simulink model "final_control_model08t02_02"  (R2014b)
settings: Solver=ode3  StartTime=0.0  StopTime=1200  FixedStep=0.1  RelTol=1e-3
libraries: simulink x2
settings Model: PauseTimes=0  SnapshotBufferSize=100  Creator=Administrator  LastModifiedBy=Administrator

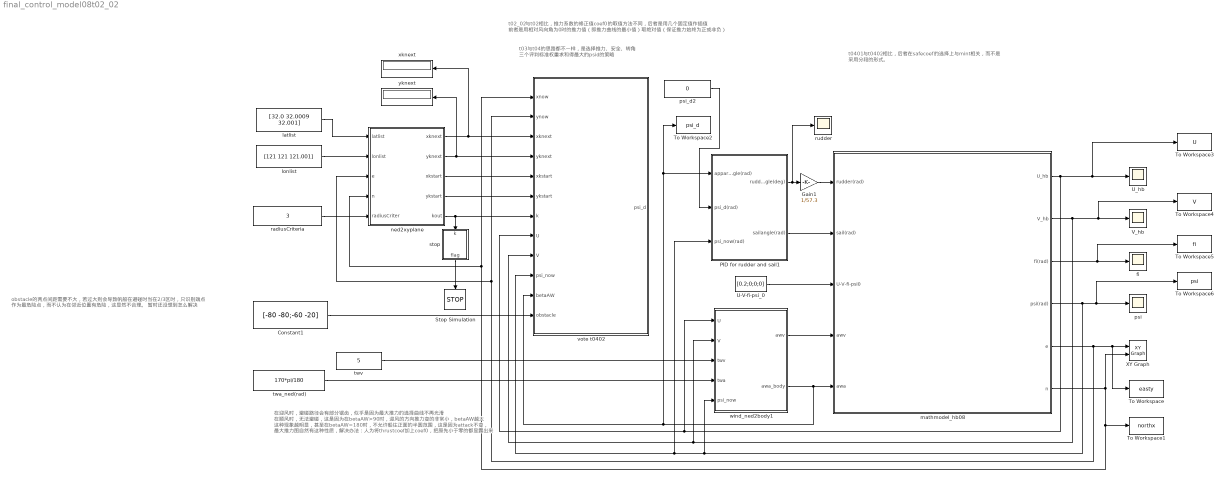
== system final_control_model08t02_02 ==
  note: obstacle的两点间距需要不大，若过大则会导致帆船在避碰时当在2/3区时，只识别端点
      | 作为最危险点，而不认为在邻近位置有危险，这显然不合理。
      | 暂时还没想到怎么解决
  note: t02_02与t02相比，推力系数的修正值coef0的取值方法不同，后者是用几个固定值作插值
      | 前者是用相对风向角为0时的推力值（即推力曲线的最小值）取绝对值（保证推力始终为正或非负）
  note: t0401与t0402相比，后者在safecoef的选择上与mint相关，而不是
      | 采用分段的形式。
  note: 在迎风时，避碰路径会有部分锯齿，似乎是因为最大推力的选择曲线不再光滑
      | 在顺风时，无法避碰，这是因为在betaAW>90时，迎风的方向推力变的非常小，betaAW越大
      | 这种现象越明显，甚至在betaAW=180时，不允许船往正面的半圆范围，这是因为attack不变，
      | 最大推力图自然有这种性质，解决办法：人为将thrustcoef加上coef0，把原先小于零的都显露出来
  note: t03与t04的思路都不一样，是选择推力、安全、转角
      | 三个评判标准权重求和得最大的psid的策略
  Constant1 : Constant  Value=[-80 -80;-60 -20]
  Gain1 : Gain  Gain=1/57.3
  PID for rudder and sail1 : Subsystem
  Stop Simulation : Stop
  To Workspace : ToWorkspace  VariableName=easty  SaveFormat=Timeseries  SampleTime=-1
  To Workspace1 : ToWorkspace  VariableName=northx  SaveFormat=Timeseries  SampleTime=-1
  To Workspace2 : ToWorkspace  VariableName=psi_d  SaveFormat=Timeseries  SampleTime=-1
  To Workspace3 : ToWorkspace  VariableName=U  SaveFormat=Timeseries  SampleTime=-1
  To Workspace4 : ToWorkspace  VariableName=V  SaveFormat=Timeseries  SampleTime=-1
  To Workspace5 : ToWorkspace  VariableName=fi  SaveFormat=Timeseries  SampleTime=-1
  To Workspace6 : ToWorkspace  VariableName=psi  SaveFormat=Timeseries  SampleTime=-1
  U-V-fi-psi_0 : Constant  Value=[0.2;0;0;0]
  U_hb : Scope
      settings: YMin=-0.045  YMax=0  SaveName=ScopeData2
  V_hb : Scope
      settings: YMin=-0.1  YMax=0.1
  XY Graph : simulink/Sinks/XY Graph  xmin=-050  xmax=150  ymin=-50  ymax=150  st=-1
  fi : Scope
      settings: YMin=-0.2  YMax=0.25
  "latlist " : Constant  Value=[32.0 32.0009 32.001]
  lonlist : Constant  Value=[121 121 121.001]
  "mathmodel_hb08 " : Subsystem
  ned2xyplane : Subsystem
  "psi " : Scope
      settings: YMin=-4  YMax=4  SaveName=ScopeData3
  psi_d2 : Constant  Value=0
  radiusCriteria : Constant  Value=3
  rudder : Scope
      settings: YMin=-40  YMax=40  SaveName=ScopeData4
  stop : MATLAB Function  TreatAsAtomicUnit=on
  twa_ned(rad) : Constant  Value=170*pi/180
  twv : Constant  Value=5
  vote t0402 : MATLAB Function  TreatAsAtomicUnit=on
  wind_ned2body1 : Subsystem
  xknext : Display
  yknext : Display
  wires:
  U-V-fi-psi_0/1 -> "mathmodel_hb08 "/3(U-V-fi-psi0)
  "mathmodel_hb08 "/1(U_hb) -> To Workspace3/1, U_hb/1, vote t0402/8(U), wind_ned2body1/1(U)
  "mathmodel_hb08 "/2(V_hb) -> vote t0402/9(V), wind_ned2body1/2(V), To Workspace4/1, V_hb/1
  "mathmodel_hb08 "/3(fi(rad)) -> To Workspace5/1, fi/1
  "mathmodel_hb08 "/4(psi(rad)) -> To Workspace6/1, "psi "/1, PID for rudder and sail1/3(psi_now(rad)), vote t0402/10(psi_now), wind_ned2body1/5(psi_now)
  PID for rudder and sail1/1(rudderangle(deg)) -> rudder/1, Gain1/1
  PID for rudder and sail1/2(sailangle(rad)) -> "mathmodel_hb08 "/2(sail(rad))
  Gain1/1 -> "mathmodel_hb08 "/1(rudder(rad))
  "mathmodel_hb08 "/5(e) -> To Workspace/1, XY Graph/1, vote t0402/2(ynow), ned2xyplane/3(e)
  "mathmodel_hb08 "/6(n) -> To Workspace1/1, ned2xyplane/4(n), vote t0402/1(xnow), XY Graph/2
  wind_ned2body1/2(awa_body) -> "mathmodel_hb08 "/5(awa), To Workspace2/1, PID for rudder and sail1/1(apparent wind angle(rad)), vote t0402/11(betaAW)
  wind_ned2body1/1(awv) -> "mathmodel_hb08 "/4(awv)
  twv/1 -> wind_ned2body1/3(twv)
  twa_ned(rad)/1 -> wind_ned2body1/4(twa)
  Constant1/1 -> vote t0402/12(obstacle)
  ned2xyplane/2(yknext) -> yknext/1, vote t0402/4(yknext)
  ned2xyplane/1(xknext) -> xknext/1, vote t0402/3(xknext)
  "latlist "/1 -> ned2xyplane/1(latlist)
  lonlist/1 -> ned2xyplane/2(lonlist)
  radiusCriteria/1 -> ned2xyplane/5(radiusCriter)
  ned2xyplane/3(xkstart) -> vote t0402/5(xkstart)
  ned2xyplane/4(ykstart) -> vote t0402/6(ykstart)
  ned2xyplane/5(kout) -> stop/1(k), vote t0402/7(k)
  stop/1(flag) -> Stop Simulation/1
  psi_d2/1 -> PID for rudder and sail1/2(psi_d(rad))

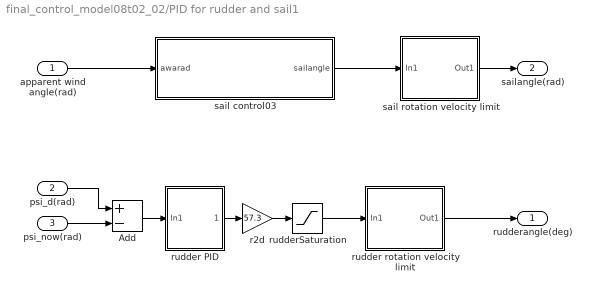
== system final_control_model08t02_02/PID for rudder and sail1 ==
  apparent wind angle(rad) : Inport
  psi_d(rad) : Inport  Port=2
  psi_now(rad) : Inport  Port=3
  Add : Sum  Inputs=+-
  r2d : Gain  Gain=57.3
  rudder PID : Subsystem
  rudder rotation velocity limit : Subsystem
  rudderSaturation : Saturate  UpperLimit=35  LowerLimit=-35
  sail control03 : MATLAB Function  TreatAsAtomicUnit=on
  sail rotation velocity limit : Subsystem
  rudderangle(deg) : Outport
  sailangle(rad) : Outport  Port=2
  wires:
  apparent wind angle(rad)/1 -> sail control03/1(awarad)
  psi_now(rad)/1 -> Add/2
  psi_d(rad)/1 -> Add/1
  Add/1 -> rudder PID/1(In1)
  rudder PID/1(rudder) -> r2d/1
  r2d/1 -> rudderSaturation/1
  rudderSaturation/1 -> rudder rotation velocity limit/1(In1)
  rudder rotation velocity limit/1(Out1) -> rudderangle(deg)/1
  sail control03/1(sailangle) -> sail rotation velocity limit/1(In1)
  sail rotation velocity limit/1(Out1) -> sailangle(rad)/1

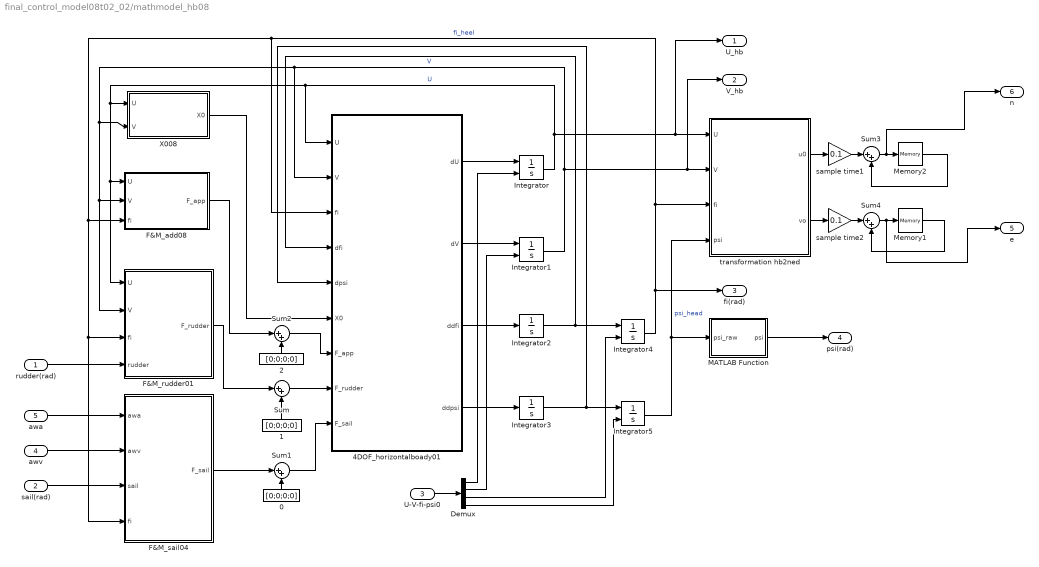
== system final_control_model08t02_02/mathmodel_hb08  ==
  rudder(rad) : Inport
  sail(rad) : Inport  Port=2
  U-V-fi-psi0 : Inport  Port=3
  awv : Inport  Port=4
  awa : Inport  Port=5
  0 : Constant  Value=[0;0;0;0]
  1 : Constant  Value=[0;0;0;0]
  2 : Constant  Value=[0;0;0;0]
  4DOF_horizontalboady01 : MATLAB Function  TreatAsAtomicUnit=on
  Demux : Demux
  F&M_add08 : MATLAB Function  TreatAsAtomicUnit=on
  F&M_rudder01 : MATLAB Function  TreatAsAtomicUnit=on
  F&M_sail04 : MATLAB Function  TreatAsAtomicUnit=on
  Integrator{,1,4..5} (4 alike) : Integrator  InitialConditionSource=external
  Integrator2 : Integrator
  Integrator3 : Integrator
  MATLAB Function : MATLAB Function  TreatAsAtomicUnit=on
  Memory1 : Memory  InheritSampleTime=on
  Memory2 : Memory  InheritSampleTime=on
  Sum{,1..4} (5 alike) : Sum  Inputs=|++
  X008 : MATLAB Function  TreatAsAtomicUnit=on
  sample time1 : Gain  Gain=0.1
  sample time2 : Gain  Gain=0.1
  transformation hb2ned : MATLAB Function  TreatAsAtomicUnit=on
  U_hb : Outport
  V_hb : Outport  Port=2
  fi(rad) : Outport  Port=3
  psi(rad) : Outport  Port=4
  e : Outport  Port=5
  n : Outport  Port=6
  wires:
  Integrator2/1 -> Integrator4/1, 4DOF_horizontalboady01/4(dfi)
  Integrator4/1 -> fi(rad)/1, transformation hb2ned/3(fi), 4DOF_horizontalboady01/3(fi), F&M_add08/3(fi), F&M_rudder01/3(fi), F&M_sail04/4(fi)  "fi_heel"
  4DOF_horizontalboady01/2(dV) -> Integrator1/1
  Integrator3/1 -> Integrator5/1, 4DOF_horizontalboady01/5(dpsi)
  4DOF_horizontalboady01/3(ddfi) -> Integrator2/1
  Integrator5/1 -> transformation hb2ned/4(psi), MATLAB Function/1(psi_raw)  "psi_head"
  X008/1(X0) -> 4DOF_horizontalboady01/6(X0)
  4DOF_horizontalboady01/1(dU) -> Integrator/1
  4DOF_horizontalboady01/4(ddpsi) -> Integrator3/1
  Integrator/1 -> 4DOF_horizontalboady01/1(U), F&M_add08/1(U), F&M_rudder01/1(U), X008/1(U), U_hb/1, transformation hb2ned/1(U)  "U"
  Integrator1/1 -> F&M_add08/2(V), F&M_rudder01/2(V), X008/2(V), 4DOF_horizontalboady01/2(V), V_hb/1, transformation hb2ned/2(V)  "V"
  Demux/3 -> Integrator4/2
  awa/1 -> F&M_sail04/1(awa)
  Demux/1 -> Integrator/2
  sail(rad)/1 -> F&M_sail04/3(sail)
  awv/1 -> F&M_sail04/2(awv)
  rudder(rad)/1 -> F&M_rudder01/4(rudder)
  Demux/4 -> Integrator5/2
  Demux/2 -> Integrator1/2
  F&M_rudder01/1(F_rudder) -> Sum/1
  F&M_add08/1(F_app) -> Sum2/1
  sample time2/1 -> Sum4/1
  Sum3/1 -> Memory2/1, n/1
  Memory2/1 -> Sum3/2
  F&M_sail04/1(F_sail) -> Sum1/1
  Sum2/1 -> 4DOF_horizontalboady01/7(F_app)
  transformation hb2ned/2(vo) -> sample time2/1
  Memory1/1 -> Sum4/2
  Sum4/1 -> e/1, Memory1/1
  U-V-fi-psi0/1 -> Demux/1
  2/1 -> Sum2/2
  Sum/1 -> 4DOF_horizontalboady01/8(F_rudder)
  sample time1/1 -> Sum3/1
  1/1 -> Sum/2
  0/1 -> Sum1/2
  transformation hb2ned/1(u0) -> sample time1/1
  Sum1/1 -> 4DOF_horizontalboady01/9(F_sail)
  MATLAB Function/1(psi) -> psi(rad)/1

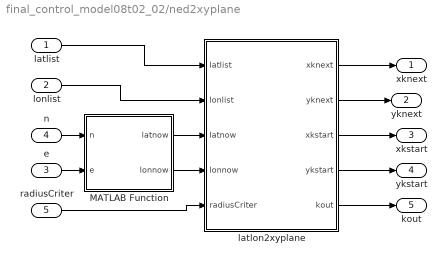
== system final_control_model08t02_02/ned2xyplane ==
  latlist : Inport
  lonlist : Inport  Port=2
  e : Inport  Port=3
  n : Inport  Port=4
  radiusCriter : Inport  Port=5
  MATLAB Function : MATLAB Function  TreatAsAtomicUnit=on
  latlon2xyplane : MATLAB Function  TreatAsAtomicUnit=on
  xknext : Outport
  yknext : Outport  Port=2
  xkstart : Outport  Port=3
  ykstart : Outport  Port=4
  kout : Outport  Port=5
  wires:
  latlon2xyplane/2(yknext) -> yknext/1
  latlist/1 -> latlon2xyplane/1(latlist)
  lonlist/1 -> latlon2xyplane/2(lonlist)
  MATLAB Function/1(latnow) -> latlon2xyplane/3(latnow)
  latlon2xyplane/1(xknext) -> xknext/1
  radiusCriter/1 -> latlon2xyplane/5(radiusCriter)
  latlon2xyplane/3(xkstart) -> xkstart/1
  latlon2xyplane/4(ykstart) -> ykstart/1
  latlon2xyplane/5(kout) -> kout/1
  MATLAB Function/2(lonnow) -> latlon2xyplane/4(lonnow)
  e/1 -> MATLAB Function/2(e)
  n/1 -> MATLAB Function/1(n)

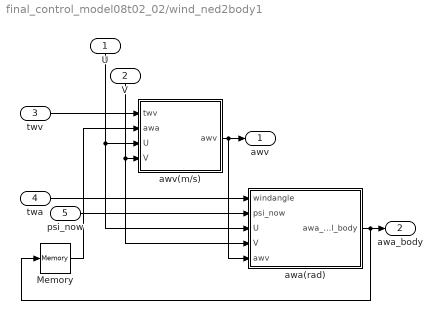
== system final_control_model08t02_02/wind_ned2body1 ==
  U : Inport
  V : Inport  Port=2
  twv : Inport  Port=3
  twa : Inport  Port=4
  psi_now : Inport  Port=5
  Memory : Memory
  awa(rad) : MATLAB Function  TreatAsAtomicUnit=on
  awv(m/s) : MATLAB Function  TreatAsAtomicUnit=on
  awv : Outport
  awa_body : Outport  Port=2
  wires:
  twa/1 -> awa(rad)/1(windangle)
  Memory/1 -> awv(m/s)/2(awa)
  twv/1 -> awv(m/s)/1(twv)
  V/1 -> awa(rad)/4(V), awv(m/s)/4(V)
  awv(m/s)/1(awv) -> awa(rad)/5(awv), awv/1
  psi_now/1 -> awa(rad)/2(psi_now)
  U/1 -> awa(rad)/3(U), awv(m/s)/3(U)
  awa(rad)/1(awa_cal_body) -> Memory/1, awa_body/1

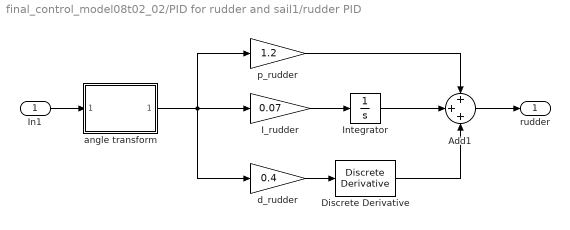
== system final_control_model08t02_02/PID for rudder and sail1/rudder PID ==
  In1 : Inport
  Add1 : Sum  Inputs=+++
  Discrete Derivative : simulink/Discrete/Discrete Derivative  gainval=1.0  ICPrevScaledInput=0.0  InputProcessing=Inherited  OutMin=[]  OutMax=[]  OutDataType=fixdt(1, 16)  OutScaling=2^-10  DoSatur=off
  I_rudder : Gain  Gain=0.07
  Integrator : Integrator
  angle transform : MATLAB Function  TreatAsAtomicUnit=on
  d_rudder : Gain  Gain=0.4
  p_rudder : Gain  Gain=1.2
  rudder : Outport
  wires:
  Integrator/1 -> Add1/2
  Discrete Derivative/1 -> Add1/3
  p_rudder/1 -> Add1/1
  d_rudder/1 -> Discrete Derivative/1
  angle transform/1(delta_pid) -> p_rudder/1, d_rudder/1, I_rudder/1
  In1/1 -> angle transform/1(delta_psi)
  I_rudder/1 -> Integrator/1
  Add1/1 -> rudder/1

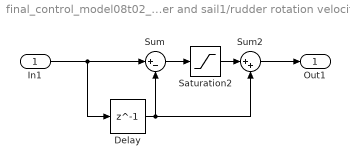
== system final_control_model08t02_02/PID for rudder and sail1/rudder rotation velocity limit ==
  In1 : Inport
  Delay : Delay  DelayLength=1  InitialCondition=0
  Saturation2 : Saturate  UpperLimit=4  LowerLimit=-4
  Sum : Sum  Inputs=|+-
  Sum2 : Sum  Inputs=|++
  Out1 : Outport
  wires:
  In1/1 -> Delay/1, Sum/1
  Sum2/1 -> Out1/1
  Saturation2/1 -> Sum2/1
  Sum/1 -> Saturation2/1
  Delay/1 -> Sum/2, Sum2/2

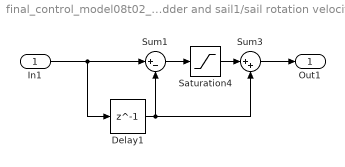
== system final_control_model08t02_02/PID for rudder and sail1/sail rotation velocity limit ==
  In1 : Inport
  Delay1 : Delay  DelayLength=1  InitialCondition=0
  Saturation4 : Saturate  UpperLimit=4  LowerLimit=-4
  Sum1 : Sum  Inputs=|+-
  Sum3 : Sum  Inputs=|++
  Out1 : Outport
  wires:
  In1/1 -> Sum1/1, Delay1/1
  Saturation4/1 -> Sum3/1
  Sum3/1 -> Out1/1
  Sum1/1 -> Saturation4/1
  Delay1/1 -> Sum3/2, Sum1/2

== matlab function final_control_model08t02_02/wind_ned2body1/awa(rad) ==
  data: windangle input; awa_cal_body output; psi_now input; U input; V input; awv input
function awa_cal_body = fcn(windangle,psi_now,U,V,awv)
%#codegen
%calculate instead of real awa in sailboat
%the wind directi is defined as common,the wind of north means the windangle is 0
Vyacht = sqrt(U^2 + V^2);
leeway = atan2( V , U);
windangle=mod(windangle,2*pi);
if windangle>pi
    windangle=windangle-2*pi;
end
%now the windangle[-pi,pi) and is defined as regular
%psi_now(-pi,pi)
twa_cal_body=mod(windangle-psi_now,2*pi);
if twa_cal_body>pi
    twa_cal_body=-2*pi+twa_cal_body;
end
asinvalue = Vyacht*sin(twa_cal_body - leeway)/awv;
if  asinvalue > 1
     asinvalue = 1;
elseif asinvalue < -1;
    asinvalue = -1;
end
awa_cal_body = twa_cal_body - asin(asinvalue);
end

== matlab function final_control_model08t02_02/ned2xyplane/MATLAB Function ==
  data: n input; latnow output; e input; lonnow output
function [latnow , lonnow] = fcn(n , e)
%#codegen
radiusEarth = 6378000;
latnow = 32 + n*180/pi/radiusEarth;
lonnow = 121 + e*180/pi/radiusEarth/cos(n/radiusEarth);

== matlab function final_control_model08t02_02/PID for rudder and sail1/rudder PID/angle transform ==
  data: delta_psi input; delta_pid output
function delta_pid = fcn(delta_psi)
%#codegen
if delta_psi > pi
    delta_pid = mod(delta_psi,2*pi) - 2*pi;
elseif delta_psi < -pi
    delta_pid = mod(delta_psi,2*pi);
else
    delta_pid = delta_psi;
end

== matlab function final_control_model08t02_02/mathmodel_hb08 /F&M_add08 ==
  data: par parameter; F_app output; U input; V input; fi input
function F_app = fcn(par,U,V,fi)
%引用的是predicting the speed of sailing
%yachts的附录3的回归公式，是针对IACC美洲杯竞技船的船模试验结果，虽然船型有些不一致，但是作为近似结果已经足够且合适。
F_app=zeros(4,1);
Vyacht = sqrt(U^2 + V^2);
q=0.5*par.rouwater*Vyacht^2*(par.swet*0.7/2+par.areakeel);
%似乎因横倾产生的增阻乘的是船体湿表面积，诱导阻力和因leeway产生的增阻才乘area_LT侧向面积？此处为方便计做了任！性！简化
%sail(angle) is positive when the sail trailing is on the starboard(righthand)(-pi,pi)
leeway=atan2(V,U);
Fn = Vyacht/sqrt(par.g*par.lwl);
sideForce_TH = q*cos(fi)*coef_LTH( fi , leeway , Fn );
resistAdd_TH = q*coef_RTH1( fi , leeway , Fn ); 
sideForce_Y = sideForce_TH*cos(leeway) - resistAdd_TH*sin(leeway);
resistAdd_X = -resistAdd_TH*cos(leeway)-sideForce_TH*sin(leeway); 

F_app(1) = resistAdd_X;
F_app(2) = sideForce_Y;
F_app(3) = sideForce_Y*cos(fi)*par.zsf;
F_app(4) = resistAdd_X*par.zsf*sin(fi) + sideForce_Y*par.xsf;
% moment_N=Mb*sin(fi)+Nb*cos(fi)
end
function coef = coef_LTH( fi , beta , Fn )
% 当漂角为我定义的正时（U>0,V>0),coef_LTH<0;反之为正
    attackHull = abs(beta*cos(fi));
    coef = -0.07092*fi^2 + 1.649*(1 - 0.2321*fi^2)*attackHull + 0.4534*attackHull^2 - 39.31*fi*Fn*attackHull^3;
    if beta > 0
        coef = -coef;
    end           
end

function coef = coef_RTH1( fi , beta , Fn )
% 基本coef_RTH1为正，所以注意作为阻力项需要另加负号
    beta = abs(beta);
    attackHull = beta*cos(fi);
    coef_LaTH = -0.07092*fi^2 + 1.649*(1 - 0.2321*fi^2)*attackHull;
    ARe = 8*pi*(1.649*(1-0.2321*fi^2))/(4*pi^2 - (1.649*(1-0.2321*fi^2))^2);
    if attackHull > 0.15
        coef = 0.002319*abs(fi) + 0.3501*fi^2*Fn^4 + (0.8141 + 5.47*Fn^2)*(coef_LaTH^2/(pi*ARe)) + 74.9*(attackHull - 0.15)^3;
    else
        coef = 0.002319*abs(fi) + 0.3501*fi^2*Fn^4 + (0.8141 + 5.47*Fn^2)*(coef_LaTH^2/(pi*ARe));
    end
end

== matlab function final_control_model08t02_02/stop ==
  data: k input; flag output
function flag = fcn(k)
%#codegen
if k == 2
    flag = 1;
else
    flag = 0;
end

== matlab function final_control_model08t02_02/ned2xyplane/latlon2xyplane ==
  data: latlist input; lonlist input; latnow input; lonnow input; xknext output; yknext output; radiusCriter input; xkstart output; ykstart output; kout output
function [ xknext , yknext , xkstart , ykstart , kout] = fcn(latlist , lonlist , latnow , lonnow , radiusCriter)
% lat/lon全是角度制数
persistent k
if isempty(k)
    k = 0;
end
num_path=min(length(latlist),length(lonlist));
if k >= num_path
   k = num_path;
   latnext = latlist(k);
   lonnext = lonlist(k);
   latstart = latnow;
   lonstart = lonnow;
else
    if k == 0      
        latstart = latnow;
        lonstart = lonnow;
    else
        latstart = latlist(k);
        lonstart = lonlist(k);
    end
   latnext = latlist(k+1);
   lonnext = lonlist(k+1);
end
[xnow , ynow]  = latlon2xy(latnow , lonnow);
[xkstart , ykstart] = latlon2xy(latstart , lonstart);
[xknext , yknext] = latlon2xy(latnext , lonnext);
delta_x = xknext - xkstart;
delta_y = yknext - ykstart;

if delta_x==0 && delta_y==0
    along_s = 0;
    cross_e = 0;
    k = k+1;
else
    alphak=atan2(yknext - ykstart , xknext - xkstart);
    cross_e=[-sin(alphak),cos(alphak)]*[xnow - xkstart;ynow - ykstart];
    along_s=[cos(alphak),sin(alphak)]*[xnow - xkstart;ynow - ykstart];    
    along_k=sqrt(delta_x^2+delta_y^2);
    if sqrt((xnow - xknext)^2+(ynow - yknext)^2) <= radiusCriter %|| along_k - along_s <= 0.5*radiusCriter
        k = k + 1;
    end    
end
kout = k;
end

function [x , y] = latlon2xy(lat , lon)    
% lat lon均是角度制,x北y东z地坐标系
radiusEarth = 6378000;
x = radiusEarth*(lat-32)*pi/180;
y = radiusEarth*cos((lat-32)*pi/180)*(lon-121)*pi/180;
end

== matlab function final_control_model08t02_02/PID for rudder and sail1/sail control03 ==
  data: awarad input; sailangle output
function sailangle = fcn(awarad)
%#codegen
beta_awdata = [0:10:180]*pi/180;
attackdata = [0 8 8 8 8 27 31 39 39 50 50 55 59 64 64 73 77 82 90]*pi/180;
% attackdata = [0 10 10 10 10 10 10 10 10 30 30 30 30 30 30 30 30 30 30]*pi/180;
awarad = mod(awarad,2*pi);
if awarad > pi
    awarad = awarad - 2*pi;
end
if awarad >= 0
    k = -1;
else
    k = 1;
end
saildata = beta_awdata - attackdata; %[0 2 12 22 32 23 29 31 41 40 50 55 61 66 76 77 83 88 90]
sailangle = k*interp1(beta_awdata , saildata , abs(awarad));

== matlab function final_control_model08t02_02/vote t0402 ==
  data: xnow input; psi_d output; ynow input; xknext input; yknext input; xkstart input; ykstart input; k input; U input; V input; psi_now input; betaAW input; obstacle input
function psi_d  = fcn(xnow , ynow , xknext , yknext , xkstart , ykstart , k , U , V , psi_now , betaAW , obstacle )
% obstacle为障碍物相对xk,yk的形状位置(限定为仅有一个多边形，若有多个障碍物设想（但此处未实现）可以在相邻探测点发现无障碍点的出现)
numvert = size(obstacle , 2);
xobstacle = zeros(1 , numvert);
yobstacle = zeros(1 , numvert);
for i = 1 : numvert
    xobstacle(i) = xkstart + obstacle(1,i);
    yobstacle(i) = ykstart + obstacle(2,i);
end

betaLeeway = atan2(V , U);
psiTarget = atan2(yknext - ynow ,xknext - xnow);
lengthb2t = sqrt((xknext - xnow)^2 + (yknext - ynow)^2);

pc = [50 30 150]; % pc = [50 30 150]; %对于顺风时需要大一点的pc，所以这样设计
ntack = howntack(xknext , yknext , xkstart , ykstart , psi_now , betaAW ,  lengthb2t , pc);
ntackam1 = 1.0; %这个系数是对ntack的修正，当遇到障碍物时，加大ntack，以防止船因为考虑ntack而走不出来
ntackam2 = 1.0;

thrustRightmax = 0;
psi_dRight = psi_now;
for deltaalpha = 0 : 5*pi/180 : 180*pi/180
    betaD = betaAW + deltaalpha;
    thrustCoef = thrust4psid(betaD , betaAW);
    psiD = betaD + psi_now;
    if k == 0 || k == 1
        safeCoef = avoidance(psiD , xnow , ynow , xobstacle , yobstacle);
    else
        safeCoef = 1;
    end
    thrustRight = safeCoef*thrustCoef*[cos(psiD),sin(psiD)]*[cos(psiTarget),sin(psiTarget)]';
    if thrustRight > thrustRightmax
        thrustRightmax = thrustRight;
        psi_dRight = psiD;
        if safeCoef < 0.5
            ntackam1 = 1.5;
        else
            ntackam1 = 1.0;
        end
    end
end
thrustLeftmax = 0;
psi_dLeft = psi_now;
for deltaalpha = 0 : 5*pi/180 : 180*pi/180
    betaD = betaAW - deltaalpha;
    thrustCoef = thrust4psid(betaD , betaAW);
    psiD = betaD + psi_now;
    if k == 0 || k == 1
        safeCoef = avoidance(psiD , xnow , ynow , xobstacle , yobstacle);
    else
        safeCoef = 1;
    end
    thrustLeft = safeCoef*thrustCoef*[cos(psiD),sin(psiD)]*[cos(psiTarget),sin(psiTarget)]';
    if thrustLeft > thrustLeftmax
        thrustLeftmax = thrustLeft;
        psi_dLeft = psiD;
        if safeCoef < 0.5
            ntackam2 = 1.5;
        else
            ntackam2 = 1.0;
        end
    end
end

ntackam = max(ntackam1 , ntackam2);
deltamaxRight = mod(abs(psi_dRight - psi_now),2*pi);
if deltamaxRight > pi
    deltamaxRight = deltamaxRight - 2*pi;
end
deltamaxLeft = mod(abs(psi_dLeft - psi_now),2*pi);
if deltamaxLeft > pi
    deltamaxLeft = deltamaxLeft - 2*pi;
end

if abs(deltamaxRight) < abs(deltamaxLeft)
    if thrustLeftmax > ntackam*ntack*thrustRightmax
        psi_d = psi_dLeft;
    else
        psi_d = psi_dRight;
    end
else
    if thrustRightmax > ntackam*ntack*thrustLeftmax
        psi_d = psi_dRight;
    else
        psi_d = psi_dLeft;
    end
end
end

function thrustCoef = thrust4psid(betaD , betaAW)
    arsail = 2.5;
    attack = howcontrolsail(betaAW);
    if abs(attack) > 10
        attack = 10;
    end
    [cls,cds] = sailcoef(attack,arsail);
    theta = atan(cds/cls);
    alpha = mod(betaD - betaAW , 2*pi);
    if alpha > pi
        alpha = alpha - 2*pi;
        k = -1;
    else
        k = 1;
    end
    if abs(betaAW) >= 140*pi/180
        coef0 = abs(sqrt(cls^2+cds^2)*sin(theta));
         % 对于正顺和侧顺时，由于最大推力曲线的图形特性，有很大程度可行方向都被舍弃，因此人为加上coef0来避免这个现象
    else
        coef0 = 0;
    end
    if alpha < 0 
        thrustCoef = k*sqrt(cls^2+cds^2)*sin(alpha + theta) + coef0;
    elseif alpha > 0
        thrustCoef = k*sqrt(cls^2+cds^2)*sin(alpha - theta) + coef0;
    else
        thrustCoef = 0;
    end
    if thrustCoef < 0
        thrustCoef = 0;
    end
end

function attack = howcontrolsail(betaAW)
    betaAW = mod(betaAW,2*pi);
    if betaAW > pi
        betaAW = betaAW - 2*pi;
        k = -1;
    else
        k = 1;
    end
    betaAWdata = [0:10:180]*pi/180;
    attackdata = [8 8 8 8 8 27 31 39 39 50 50 55 59 64 64 73 77 82 90]*pi/180;
    attack = k*interp1(betaAWdata , attackdata , abs(betaAW));
end

function [Cls,Cds] = sailcoef(attack,arsail)
% generate a lookup table for the lift/drag coefficients for the sail
% and compute Cls/Cds from the lookup table using interpolation.
% lookup table
adata =pi/180*[0	1	2	3	4	5	6	7	8	9	10	11	12	13	14	15	16 ...
    17	18	19	20	21	22	23	24	25	26	27	30	35	40	45	50	55	60 ...
    65	70	75	80	85	90	95	100	105	110	115	120	125	130	135	140	145	150 ...
    155	160	165	170	175	180];
cldata = [0.0000	0.1100	0.2200	0.3300	0.4180	0.5180	0.5048	0.6760	0.7189...
    0.6969	0.5122	0.1642	0.0749	0.0967	0.1382	0.1861	0.2364	0.2873...
    0.3393	0.3927	0.4463	0.5001	0.5539	0.6078	0.6617	0.7156	0.7700...
    0.8277	0.8550	0.9800	1.0350	1.0500	1.0200	0.9550	0.8750	0.7600...
    0.6300	0.5000	0.3650	0.2300	0.0900	-0.0500	-0.1850	-0.3200	-0.4500...
    -0.5750	-0.6700	-0.7600	-0.8500	-0.9300	-0.9800	-0.9000	-0.7700	-0.6700...
    -0.6350	-0.6800	-0.8500	-0.6600	0.0000];
cddata = [0.0147	0.0148	0.0151	0.0156	0.0168	0.0181	0.0197	0.0214	0.0234...
    0.0255	0.0277	0.0760	0.1230	0.1400	0.1580	0.1770	0.1960	0.2170...
    0.2380	0.2600	0.2820	0.3050	0.3290	0.3540	0.3790	0.4050	0.4320...
    0.4600	0.5700	0.7450	0.9200	1.0750	1.2150	1.3450	1.4700	1.5750...
    1.6650	1.7350	1.7800	1.8000	1.8000	1.7800	1.7500	1.7000	1.6350...
    1.5550	1.4650	1.3500	1.2250	1.0850	0.9250	0.7550	0.5750	0.4200...
    0.3200	0.2300	0.1400	0.0550	0.0250];
% 展弦比换算
xdata = adata + cldata./pi*(1/arsail);
yldata = cldata;
yddata = cddata + cldata.^2/pi*(1/arsail);
[xdata , xnum] = sort(xdata);
yldata = yldata(xnum);
yddata = yddata(xnum);

attack=mod(attack,2*pi);
if attack>pi
    attack=attack-2*pi;
end

if attack>=0
    Cls = interp1(xdata,yldata,attack);
    Cds = interp1(xdata,yddata,attack);
else
    Cls = -1*interp1(xdata,yldata,-attack);
    Cds = interp1(xdata,yddata,-attack);
end
end

function safeCoef = avoidance(psiD , xnow , ynow , xobstacle , yobstacle )
% obstacle需要按照边界顺序罗列
Lmax = 50;
numvert = size(xobstacle , 2);
if numvert == 2
    obstyle = 'line';
elseif numvert <= 1 
    obstyle = 'point';
else
    obstyle = 'polygon';
end

if strcmp(obstyle,'line')
    vert1 = [xobstacle(1),yobstacle(1)];
    vert2 = [xobstacle(2),yobstacle(2)];
    distvert12 = (vert1-vert2)*(vert1-vert2)';
    if distvert12 > 0.5*Lmax
        vert11 = (vert1 + vert2)/2;
         safeCoef1 = avoidline(psiD , xnow , ynow , vert11  , vert2);
        safeCoef2 = avoidline(psiD , xnow , ynow , vert11  , vert1);
        safeCoef = min(safeCoef1,safeCoef2);
    else
        safeCoef = avoidline(psiD , xnow , ynow , vert1  , vert2);
    end
elseif strcmp(obstyle,'polygon')
    safeCoeflist = zeros(1,numvert*(numvert-1)/2);
    k = 0;
    for i = 2 : numvert
        for j = 1 : i-1
            k = k + 1;
            vert1 = [xobstacle(i),yobstacle(i)];
            vert2 = [xobstacle(j),yobstacle(j)];
        	safeCoeflist(i) = avoidline(psiD , xnow , ynow , vert1 , vert2);
        end
    end
    safeCoef = min(safeCoeflist);
else
    safeCoef = 1;
end
end

function safei = avoidline(psiD , xnow , ynow , vert1 , vert2)
vect1 = vert1 - [xnow , ynow];
vect2 = vert2 - [xnow , ynow];
dirvec = [cos(psiD),sin(psiD)];

Lmin = 20;
Lmax = 50;
Lc = 0.5*Lmin;

field0 = multip(vect1 , dirvec)*multip(vect2 , dirvec);
field1 = vect1*dirvec';
field2 = vect2*dirvec';

if field1 <= 0 && field2 <= 0
    safei = 1;
elseif field0 <= 0
    d = abs(multip(vect1,(vert2-vert1))/sqrt((vert2-vert1)*(vert2-vert1)')) ; % 计算当前点到直线距离
    if d < Lmin
        safei = 0;
    elseif d < Lmax
        safei = (d - Lmin)/(Lmax - Lmin);
    else
        safei = 1;
    end
else
    if multip(vect1 , dirvec) <= 0 && multip(vect1 , vect2) < 0
        mint = vect2*dirvec';
        mincross = sqrt(vect2*vect2' - mint^2);
    elseif multip(vect2 , dirvec) >= 0 && multip(vect1 , vect2) < 0
        mint = vect1*dirvec';
        mincross = sqrt(vect1*vect1' - mint^2);
    elseif multip(vect2 , dirvec) >= 0 && multip(vect1 , vect2) >= 0
        mint = vect2*dirvec';
        mincross = sqrt(vect2*vect2' - mint^2);
    elseif multip(vect1 , dirvec) <= 0 && multip(vect1 , vect2) >= 0
        mint = vect1*dirvec';
        mincross = sqrt(vect1*vect1' - mint^2);
    else
        mint = 100;
        mincross = 100;
    end
    if mint > Lmax
        safei = 1;
    elseif mint <= Lmax && mint > Lmin
        safei = (mint - Lc)/(Lmax - Lc);
    else
        safei = min(mincross/Lc , (Lmin - Lc)/(Lmax - Lc));
    end
end
end

    

function ntack = howntack(xknext , yknext , xkstart , ykstart , psi_now , betaAW ,  lengthb2t , pc)
    a = [cos(psi_now + betaAW) , sin(psi_now + betaAW)];
    b = [xknext - xkstart , yknext - ykstart];
    if a*b' > 0
        i = 1;
    elseif a*b' == 0
        i = 2;
    else
        i = 3;
    end
    ntack = 1 + pc(i)/lengthb2t;
end

function multipCross = multip(rowvector1 , rowvector2)
    multipCross = rowvector1(1)*rowvector2(2) - rowvector1(2)*rowvector2(1);
end

== matlab function final_control_model08t02_02/wind_ned2body1/awv(m//s) ==
  data: twv input; awv output; awa input; U input; V input
function awv = fcn(twv , awa , U , V)
%#codegen
    leeway = atan2(V , U);
    Vyacht = sqrt(U^2 + V^2);
    awv = sqrt(Vyacht^2 +twv^2 + 2*Vyacht*twv*cos(awa - leeway));
end

== matlab function final_control_model08t02_02/mathmodel_hb08 /4DOF_horizontalboady01 ==
  data: par parameter; dU output; U input; V input; fi input; dfi input; dpsi input; dV output; ddfi output; ddpsi output; X0 input; F_app input; F_rudder input; F_sail input
function [dU,dV,ddfi,ddpsi] = fcn(par,U,V,fi,dfi,dpsi,X0,F_app,F_rudder,F_sail)
%#codegen
%horizontal body axis system, (x,y,z,U,V,W,fi_cap=fi,theta_cap=0,psi_cap=psi)
Vb=sqrt(U^2+V^2);
Xvdpsi = par.Xvdpsi*(0.5*par.rouwater*par.lwl^2*par.draftwithkeel);
Ydfi = par.Ydfi*(0.5*par.rouwater*par.lwl^2*par.draftwithkeel*Vb);
Ydpsi = par.Ydpsi*(0.5*par.rouwater*par.lwl^2*par.draftwithkeel*Vb);
Kdfi = par.Kdfi*(0.5*par.rouwater*par.lwl^2*par.draftwithkeel^2*Vb);
Ndpsi = par.Ndpsi*(0.5*par.rouwater*par.lwl^3*par.draftwithkeel*Vb);

KR = krcal(par, fi);

force_X=X0+F_app(1)+Xvdpsi*V*dpsi+F_rudder(1,1)+F_sail(1);
force_Y=F_app(2)+Ydfi*dfi+Ydpsi*dpsi+F_rudder(2,1)+F_sail(2);
moment_K=F_app(3)+Kdfi*dfi+F_rudder(3)+F_sail(3,1) - KR;
moment_N=F_app(4)+Ndpsi*dpsi+F_rudder(4,1)+F_sail(4);

dU=(force_X+(par.m+par.my*cos(fi)^2+par.mz*sin(fi)^2)*V*dpsi)/(par.m+par.mx);
dV=(force_Y-2*(par.mz-par.my)*sin(fi)*cos(fi)*V*dfi-(par.m+par.mx)*U*dpsi)...
    /(par.m+par.my*cos(fi)^2+par.mz*sin(fi)^2);
ddfi=(moment_K+((par.Iyy+par.Jyy)-(par.Izz+par.Jzz))*sin(fi)*cos(fi)*dpsi^2)/(par.Ixx+par.Jxx);
ddpsi=(moment_N-2*((par.Iyy+par.Jyy)-(par.Izz+par.Jzz))*sin(fi)*cos(fi)*dpsi*dfi)/((par.Iyy+par.Jyy)*sin(fi)^2+(par.Izz+par.Jzz)*cos(fi)^2);

end

function KR = krcal(par , phi) 
% zg是船体的实际重心在Zb轴上的位置，且以龙骨和船底的交界处为z=0点）,注意正方向向下
% mhull是包括船体、龙骨、舵（即桅杆和帆除外部分）的质量
gz0  = gzstandard(phi);
KR = gz0*(par.m)*par.g + (par.m)*par.g*(par.zgsailboat)*sin(phi*pi()/180);
% 注意上式中（mHull+mSail)即文先前所述将帆重的影响放入船整体中考虑
end

function gz0 = gzstandard(phi)
% 计算当假设船的重心在龙骨根部（船底与龙骨的交界处）时的GZ
% phi为横倾角且角度制,gz0单位为m
phi = phi*57.3;
heel = [0 10 20 30 40 50 60 70 80];
gz = 0.001*[0 35.14 69.12 100.04 127.65 153.15 170.43 179.32 174.00];
if phi < 0
    k = -1;
else
    k = 1;
end
if phi > 80
    phi = 80;
elseif phi < -80
    phi = -80;
end
gz0 = k*interp1(heel , gz , abs(phi));
end

== matlab function final_control_model08t02_02/mathmodel_hb08 /F&M_rudder01 ==
  data: par parameter; U input; V input; fi input; F_rudder output; rudder input
function F_rudder = fcn(par,U,V,fi,rudder)
%#codegen
% rudder is positive when operate the right rudder(-pi,pi)
F_rudder=zeros(4,1);
Vb = sqrt(U^2+V^2);
q=0.5*par.rouwater*(0.9*Vb)^2*par.arearudder;
%sail(angle) is positive when the sail trailing is on the starboard(righthand)(-pi,pi)
leeway=atan2(V,U);
attack_rudder=leeway+rudder;
[Clr,Cdr]=ruddercoef(attack_rudder);
Cx=Clr*cos(fi)*sin(leeway)-Cdr*cos(leeway);
Cy=-Clr*cos(fi)*cos(leeway)-Cdr*sin(leeway);

F_rudder(1)=Cx*q;
F_rudder(2)=Cy*q; 
F_rudder(3)=-q*Cy*par.rudder_zgce*cos(fi);
F_rudder(4)=(q*Cy*par.rudder_xgce+q*Cx*par.rudder_zgce*sin(fi));
% moment_N=Mb*sin(fi)+Nb*cos(fi)

function [Clr,Cdr] = ruddercoef(attack)
% generate a lookup table for the lift/drag coefficients for the rudder
% and compute Clr/Cdr from the lookup table using interpolation.
% lookup table
xdata = linspace(0,pi,91); % every 2.0 degrees
% lift curve
yldata = [0	0.1095	0.2202	0.3401	0.4599	0.5796	0.6984	0.7936	0.8804...
    0.952	0.9981	0.6289	0.6369	0.6631	0.6912	0.7478	0.8043	0.8609...
    0.9159	0.9606	1.0053	1.0375	1.0629	1.088	1.1114	1.1291	1.1398...
    1.1399	1.1312	1.1086	1.0858	1.0589	1.027	0.9872	0.9437	0.885...
    0.8259	0.7664	0.6999	0.6313	0.5627	0.4755	0.3809	0.2952	0.2132...
    0.132	0.0398	-0.06	-0.1589	-0.2532	-0.3103	-0.3812	-0.4692	-0.5347...
    -0.5988	-0.6611	-0.7177	-0.7738	-0.8313	-0.8835	-0.9321	-0.9655	-0.9991...
    -1.0342	-1.0591	-1.0732	-1.0717	-1.0596	-1.0475	-1.0243	-0.986	-0.9449...
    -0.8924	-0.8381	-0.7833	-0.7323	-0.7056	-0.6813	-0.699	-0.7302	-0.7662...
    -0.874	-0.8646	-0.8012	-0.7206	-0.6199	-0.5167	-0.4094	-0.2838	-0.1419	0];
% drag curve
yddata = [0.0083 0.0118	0.0164	0.0287	0.0418	0.0634	0.0851	0.1095	0.133...
    0.1547	0.1875	0.2766	0.2958	0.3127	0.3504	0.4099	0.4705	0.5411...
    0.6254	0.7185	0.8123	0.9009	0.9865	1.0723	1.1541	1.2256	1.2967...
    1.3676	1.4391	1.514	1.5884	1.6528	1.7052	1.7549	1.8031	1.8413...
    1.8798	1.919	1.9479	1.9754	2.0041	2.0241	2.0405	2.0595	2.0696...
    2.079	2.0799	2.076	2.0661	2.047	2.0125	1.9804	1.9527	1.9106...
    1.8728	1.843	1.8091	1.7703	1.7194	1.6718	1.626	1.5595	1.4931...
    1.4277	1.3667	1.3105	1.24	1.1589	1.0771	0.9937	0.908	0.8226...
    0.7412	0.661	0.5817	0.5076	0.4629	0.4185	0.3895	0.3661	0.3378...
    0.293	0.2487	0.2035	0.1582	0.1156	0.0794	0.0543	0.0353	0.0216	0.008];
attack=mod(attack,2*pi);
if attack>pi
    attack=attack-2*pi;
end

if attack>=0
    Clr = interp1(xdata,yldata,attack);
    Cdr = interp1(xdata,yddata,attack);
else
    Clr = -1*interp1(xdata,yldata,-attack);
    Cdr = interp1(xdata,yddata,-attack);
end

== matlab function final_control_model08t02_02/mathmodel_hb08 /F&M_sail04 ==
  data: par parameter; F_sail output; awa input; awv input; sail input; fi input
function F_sail = fcn(par,awa,awv,sail,fi)
%#codegen
%awa is positive when the wind blow to the right face of the sail(-pi,pi)
F_sail=zeros(4,1);
q=0.5*par.rouair*awv^2*par.areasail;
%sail(angle) is positive when the sail trailing is on the starboard(righthand)(-pi,pi)
attack_sail=awa+sail;
arsail = par.arsail;
[Cls,Cds]=sailcoef(attack_sail,arsail);
Cx=Cls*sin(awa)-Cds*cos(awa);
Cy=-Cls*cos(awa)-Cds*sin(awa);

F_sail(1)=Cx*cos(fi)^2*q;
F_sail(2)=Cy*cos(fi)^2*q;
F_sail(3)=-F_sail(2)*par.sail_zcg/cos(fi);
F_sail(4)=F_sail(2)*par.sail_xcg + F_sail(1)*par.sail_zcg*sin(fi);
% F_sail(4)=(q*Cy*par.sail_xgce+q*Cx*par.sail_zgce*cos(fi)*sin(fi)+q*Cx*par.sail_ygce*sin(fi)^2)*cos(fi)^2-par.msail*par.g*par.sail_xcg;
% F_sail(4)=q*Cy*par.sail_xgce;
% moment_N=Mb*sin(fi)+Nb*cos(fi)

function [Cls,Cds] = sailcoef(attack,arsail)
% generate a lookup table for the lift/drag coefficients for the sail
% and compute Cls/Cds from the lookup table using interpolation.
% lookup table
adata =pi/180*[0	1	2	3	4	5	6	7	8	9	10	11	12	13	14	15	16 ...
    17	18	19	20	21	22	23	24	25	26	27	30	35	40	45	50	55	60 ...
    65	70	75	80	85	90	95	100	105	110	115	120	125	130	135	140	145	150 ...
    155	160	165	170	175	180];
cldata = [0.0000	0.1100	0.2200	0.3300	0.4180	0.5180	0.5048	0.6760	0.7189...
    0.6969	0.5122	0.1642	0.0749	0.0967	0.1382	0.1861	0.2364	0.2873...
    0.3393	0.3927	0.4463	0.5001	0.5539	0.6078	0.6617	0.7156	0.7700...
    0.8277	0.8550	0.9800	1.0350	1.0500	1.0200	0.9550	0.8750	0.7600...
    0.6300	0.5000	0.3650	0.2300	0.0900	-0.0500	-0.1850	-0.3200	-0.4500...
    -0.5750	-0.6700	-0.7600	-0.8500	-0.9300	-0.9800	-0.9000	-0.7700	-0.6700...
    -0.6350	-0.6800	-0.8500	-0.6600	0.0000];
cddata = [0.0147	0.0148	0.0151	0.0156	0.0168	0.0181	0.0197	0.0214	0.0234...
    0.0255	0.0277	0.0760	0.1230	0.1400	0.1580	0.1770	0.1960	0.2170...
    0.2380	0.2600	0.2820	0.3050	0.3290	0.3540	0.3790	0.4050	0.4320...
    0.4600	0.5700	0.7450	0.9200	1.0750	1.2150	1.3450	1.4700	1.5750...
    1.6650	1.7350	1.7800	1.8000	1.8000	1.7800	1.7500	1.7000	1.6350...
    1.5550	1.4650	1.3500	1.2250	1.0850	0.9250	0.7550	0.5750	0.4200...
    0.3200	0.2300	0.1400	0.0550	0.0250];
% 展弦比换算
xdata = adata + cldata./pi*(1/arsail);
yldata = cldata;
yddata = cddata + cldata.^2/pi*(1/arsail);
[xdata , xnum] = sort(xdata);
yldata = yldata(xnum);
yddata = yddata(xnum);

attack=mod(attack,2*pi);
if attack>pi
    attack=attack-2*pi;
end

if attack>=0
    Cls = interp1(xdata,yldata,attack);
    Cds = interp1(xdata,yddata,attack);
else
    Cls = -1*interp1(xdata,yldata,-attack);
    Cds = interp1(xdata,yddata,-attack);
end

== matlab function final_control_model08t02_02/mathmodel_hb08 /MATLAB Function ==
  data: psi_raw input; psi output
function psi = fcn(psi_raw)
%#codegen
psi=mod(psi_raw,2*pi);
if psi>pi
    psi=psi-2*pi;
end

== matlab function final_control_model08t02_02/mathmodel_hb08 /X008 ==
  data: par parameter; U input; X0 output; V input
function X0 = resistance0(par,U,V)
%#采用maxsurf计算剩余阻力Rrhu，因为maxsurf也是用的delft船型经验公式，因此与论文一致
Vb = sqrt(U^2+V^2);
Reh = Vb * par.lwl*0.7/1.139*1e6;
cf = 0.075 / (log(Reh)-2)^2;
Rfhu = 0.5*par.rouwater*U^2*par.swet*cf;
fn = Vb/sqrt(par.g*par.lwl);
Rrhu = regressionRr(Vb);

Rek = Vb*par.ckeel/0.000014607;
cfk = 0.075 / (log(Rek)-2)^2;   
Rfku = 0.5*par.rouwater*U^2*par.swetkeel*cfk;  
kk = 2*par.tkeel/par.ckeel+60*(par.tkeel/par.ckeel)^4;
Rvku = Rfku*(1+kk);

Rer = Vb*par.crudder/0.000014607;
cfr = 0.075 / (log(Rer)-2)^2;   
Rfru = 0.5*par.rouwater*U^2*par.swetrudder*cfr;  
kr = 2*par.trudder/par.crudder+60*(par.trudder/par.crudder)^4;
Rvru = Rfru*(1+kr);

AA = chooseAA(fn);
Rrku = par.disprudder*par.rouwater*par.g*(AA(1)+AA(2)*(par.draft+par.bkeel)/par.bwl+AA(3)*(par.draft+par.zcbk)/par.dispkeel^(1/3)+AA(4)*par.disphull/par.dispkeel);

X0 = - Rfhu - Rrhu - Rvku - Rvru - Rrku;
end

function Rr = regressionRr(Vb)
    Vbdata = 0.5144*[0.0000	0.1250	0.2500	0.3750	0.5000	0.6250	0.7500	0.8750...
        1.0000	1.1250	1.2500	1.3750	1.5000	1.6250	1.7500	1.8750	2.0000...
        2.1250	2.2500	2.3750	2.5000	2.6250	2.7500	2.8750	3.0000	3.1250...
        3.2500	3.3750	3.5000	3.6250	3.7500	3.8750	4.0000	4.1250	4.2500...
        4.3750	4.5000	4.6250	4.7500	4.8750	5.0000	5.1250	5.2500];
    Rrdata = [0.1489	0.1328	0.1296	0.1370	0.1541	0.1803	0.2152	0.2586...
        0.3581	0.4624	0.5693	0.6812	0.8073	0.9472	1.1028	1.2637	1.4507...
        1.6742	2.0137	2.5649	3.2939	4.2294	5.6616	7.0974	8.4372	10.2109...
        11.3130	12.2094	13.8931	15.3105	16.6075	17.8199	18.8158	19.7752	20.6345...
        21.0878	21.6815	22.3729	23.1612	23.9365	24.4931	24.9375	26.1295];
    Rr = interp1(Vbdata,Rrdata,Vb,'linear','extrap');
end

function AA = chooseAA(fn)
    A0 = [-0.00104 -0.00550 -0.01110 -0.00713 -0.03581 -0.00470 0.00553 0.04822 0.01021];
    A1 = [0.00172 0.00597 0.01421 0.02632 0.08649 0.11592 0.07371 0.00660 0.14173];
    A2 = [0.00117 0.00390 0.00069 -0.00232 0.00999 -0.00064 0.05991 0.07048 0.06409];
    A3 = [-0.00008 -0.00009 0.00021 0.00039 0.00017 0.00035 -0.00114 -0.00035 -0.00192];
    x = [0.2 0.25 0.30 0.35 0.40 0.45 0.50 0.55 0.60];
    AA = zeros(1,4);
    AA(1) = interp1(x,A0,fn,'linear','extrap');
    AA(2) = interp1(x,A1,fn,'linear','extrap');
    AA(3) = interp1(x,A2,fn,'linear','extrap');
    AA(4) = interp1(x,A3,fn,'linear','extrap');
end

== matlab function final_control_model08t02_02/mathmodel_hb08 /transformation hb2ned ==
  data: U input; u0 output; V input; fi input; psi input; vo output
function [u0,vo]= fcn(U,V,fi,psi)
%#codegen
% transformations from {hb} to {ned}
R_b2n=[cos(psi) -sin(psi)*cos(fi) sin(psi)*sin(fi)
       sin(psi) cos(psi)*cos(fi) -cos(psi)*sin(fi)
       0        sin(fi)           cos(fi)];
R_hb2b=[1  0       0
        0 cos(fi)  sin(fi)
        0 -sin(fi) cos(fi)];
vb0=R_b2n*R_hb2b*[U;V;0];
u0=vb0(1);
vo=vb0(2);
